simulink model "Closed_Loop_VC"  (R2016b)
settings: Solver=ode1  StartTime=0  StopTime=4  FixedStep=Time_Step  MaxStep=100e-6  RelTol=1e-3
undefined symbols (not defined in the file): Lg, Rg, Sn, Time_Step
libraries: powerlib x25, GFM_Lib x6, Source_Lib x2
settings Model: Creator=Frederic_Colas  LastModifiedBy=Frederic_Colas
settings OptimizationCC: LifeSpan=inf
settings DebuggingCC: UnconnectedInputMsg=none  UnconnectedOutputMsg=none  UnconnectedLineMsg=none  SFExecutionAtInitializationDiag=none
settings HardwareCC: ProdBitPerSizeT=32  ProdBitPerPtrDiffT=32  ProdWordSize=32  ProdHWDeviceType=Specified
settings SimscapeCC: SimscapeNormalizeSystem=off

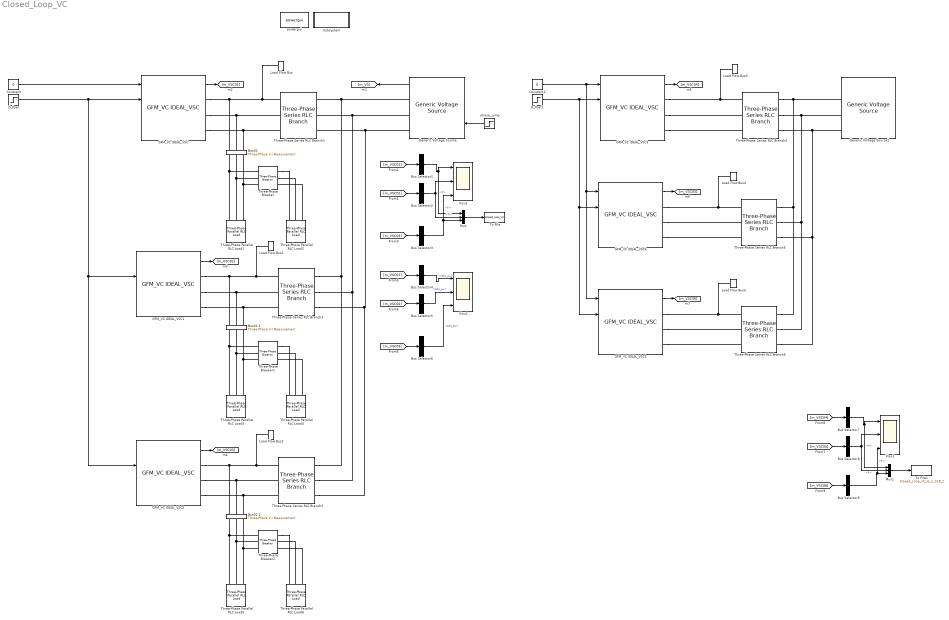
== system Closed_Loop_VC ==
  Bus Selector{1..3,7..9} (6 alike) : BusSelector  OutputSignals=P
  Bus Selector4 : BusSelector  OutputSignals=Ig.abc_pu
  Bus Selector5 : BusSelector  OutputSignals=Ig.abc_pu
  Bus Selector6 : BusSelector  OutputSignals=Ig.abc_pu
  "Bus02 " : powerlib/Measurements/Three-Phase V-I Measurement  VoltageMeasurement=no  SetLabelV=off  LabelV=Vabc  Vpu=off  VpuLL=off  CurrentMeasurement=no  SetLabelI=off  LabelI=Iabc  Ipu=off  Pbase=100e6  Vbase=500e3  OutputType=Complex  PhasorSimulation=off  PSBequivalent=0
  Bus02 1 : powerlib/Measurements/Three-Phase V-I Measurement  VoltageMeasurement=no  SetLabelV=off  LabelV=Vabc  Vpu=off  VpuLL=off  CurrentMeasurement=no  SetLabelI=off  LabelI=Iabc  Ipu=off  Pbase=100e6  Vbase=500e3  OutputType=Complex  PhasorSimulation=off  PSBequivalent=0
  Bus02 2 : powerlib/Measurements/Three-Phase V-I Measurement  VoltageMeasurement=no  SetLabelV=off  LabelV=Vabc  Vpu=off  VpuLL=off  CurrentMeasurement=no  SetLabelI=off  LabelI=Iabc  Ipu=off  Pbase=100e6  Vbase=500e3  OutputType=Complex  PhasorSimulation=off  PSBequivalent=0
  Constant : Constant  Value=0
  Constant1 : Constant  Value=0
  D_Pset : Step  Time=0.1  After=0.5  SampleTime=0
  D_Pset1 : Step  Time=0.1  After=0.5  SampleTime=0
  GFM_VC IDEAL_VSC : GFM_Lib/GFM_VC IDEAL_VSC  fn=fn  Sn=Sn  Pn=Sn  Udcn=640e3  Output_Delay=Time_Step  Un1=320e3  Un2=Un  Rt_pu=0.005  Lt_pu=0.15  Lm_pu=500  Rm_pu=500  DC_Link=Perfect DC Source  H_DC=inf  H_DC_sav=inf  wn_PLL=500  zeta_PLL=1  Val_Freq_Support=off  R_percent=4  dLc_pu=0  Rv=0.09  W_TVR=60  I_max_pu=1.2  wn_I_max=300  I_Max_TVI_pu=1.2  DX_DR=5  Advanced=off  gainpopup=Inertia Less  wn_Inertia_Less=10  Param_Inertia=PI  H_GFo=5  zeta_GFo=1  LFpopup=PQ  P0=0  Q0=0  V0=0.99839  Theta0=-0.85854
  GFM_VC IDEAL_VSC1 : GFM_Lib/GFM_VC IDEAL_VSC  fn=fn  Sn=Sn  Pn=Sn  Udcn=640e3  Output_Delay=Time_Step  Un1=320e3  Un2=Un  Rt_pu=0.005  Lt_pu=0.15  Lm_pu=500  Rm_pu=500  DC_Link=Perfect DC Source  H_DC=inf  H_DC_sav=inf  wn_PLL=50  zeta_PLL=1  Val_Freq_Support=off  R_percent=4  dLc_pu=0  Rv=0.09  W_TVR=60  I_max_pu=1.2  wn_I_max=300  I_Max_TVI_pu=1.2  DX_DR=5  Advanced=on  gainpopup=With Inertia  wn_Inertia_Less=10  Param_Inertia=VSM  H_GFo=5  zeta_GFo=1  LFpopup=PQ  P0=0  Q0=0  V0=0.99839  Theta0=-0.85854
  GFM_VC IDEAL_VSC2 : GFM_Lib/GFM_VC IDEAL_VSC  fn=fn  Sn=Sn  Pn=Sn  Udcn=640e3  Output_Delay=Time_Step  Un1=320e3  Un2=Un  Rt_pu=0.005  Lt_pu=0.15  Lm_pu=500  Rm_pu=500  DC_Link=Perfect DC Source  H_DC=inf  H_DC_sav=inf  wn_PLL=50  zeta_PLL=1  Val_Freq_Support=off  R_percent=4  dLc_pu=0  Rv=0.09  W_TVR=60  I_max_pu=1.2  wn_I_max=300  I_Max_TVI_pu=1.2  DX_DR=5  Advanced=on  gainpopup=With Inertia  wn_Inertia_Less=10  Param_Inertia=PI  H_GFo=5  zeta_GFo=1  LFpopup=PQ  P0=0  Q0=0  V0=0.99839  Theta0=-0.85854
  GFM_VC IDEAL_VSC3 : GFM_Lib/GFM_VC IDEAL_VSC  fn=fn  Sn=Sn  Pn=Sn  Udcn=640e3  Output_Delay=Time_Step  Un1=320e3  Un2=Un  Rt_pu=0.005  Lt_pu=0.15  Lm_pu=500  Rm_pu=500  DC_Link=Perfect DC Source  H_DC=inf  H_DC_sav=inf  wn_PLL=50  zeta_PLL=1  Val_Freq_Support=off  R_percent=4  dLc_pu=0  Rv=0.09  W_TVR=60  I_max_pu=1.2  wn_I_max=300  I_Max_TVI_pu=1.2  DX_DR=5  Advanced=on  gainpopup=With Inertia  wn_Inertia_Less=10  Param_Inertia=PI  H_GFo=5  zeta_GFo=1  LFpopup=PQ  P0=0  Q0=0  V0=1  Theta0=-3.2524e-13
  GFM_VC IDEAL_VSC4 : GFM_Lib/GFM_VC IDEAL_VSC  fn=fn  Sn=Sn  Pn=Sn  Udcn=640e3  Output_Delay=Time_Step  Un1=320e3  Un2=Un  Rt_pu=0.005  Lt_pu=0.15  Lm_pu=500  Rm_pu=500  DC_Link=Perfect DC Source  H_DC=inf  H_DC_sav=inf  wn_PLL=50  zeta_PLL=1  Val_Freq_Support=off  R_percent=4  dLc_pu=0  Rv=0.09  W_TVR=60  I_max_pu=1.2  wn_I_max=300  I_Max_TVI_pu=1.2  DX_DR=5  Advanced=on  gainpopup=With Inertia  wn_Inertia_Less=10  Param_Inertia=PI  H_GFo=1  zeta_GFo=1  LFpopup=PQ  P0=0  Q0=0  V0=1  Theta0=2.2332e-14
  GFM_VC IDEAL_VSC5 : GFM_Lib/GFM_VC IDEAL_VSC  fn=fn  Sn=Sn  Pn=Sn  Udcn=640e3  Output_Delay=Time_Step  Un1=320e3  Un2=Un  Rt_pu=0.005  Lt_pu=0.15  Lm_pu=500  Rm_pu=500  DC_Link=Perfect DC Source  H_DC=inf  H_DC_sav=inf  wn_PLL=50  zeta_PLL=1  Val_Freq_Support=off  R_percent=4  dLc_pu=0  Rv=0.09  W_TVR=60  I_max_pu=1.2  wn_I_max=300  I_Max_TVI_pu=1.2  DX_DR=5  Advanced=on  gainpopup=With Inertia  wn_Inertia_Less=10  Param_Inertia=PI  H_GFo=5  zeta_GFo=1  LFpopup=PQ  P0=0  Q0=0  V0=1  Theta0=2.2332e-14
  Generic Voltage Source : Source_Lib/Generic Voltage Source  SourceNature_str=INFINITE  fn=50  Sn=1e9  Un=400e3  H_s=5  DroopOnOff=on  R_percent=4  TN=1  TD=2  Time_Step=Time_Step  LFpopup=Swing  P0=898928563.4489  Q0=13470900.4169  V0=1  Theta0=0
  Generic Voltage Source1 : Source_Lib/Generic Voltage Source  SourceNature_str=INFINITE  fn=50  Sn=1e9  Un=400e3  H_s=5  DroopOnOff=on  R_percent=4  TN=1  TD=2  Time_Step=Time_Step  LFpopup=Swing  P0=3.3307e-06  Q0=7.1054e-06  V0=1  Theta0=0
  Load Flow Bus : powerlib/Measurements/Load Flow Bus  LConnTagsString=a  Phases=single  Connectors=on one side  ID=BUS_1  Vbase=400e3  Vref=1  Vangle=0  VLF=0.9984  VLFb=1  VLFc=1  angleLF=-0.8585  angleLFb=0  angleLFc=0
  Load Flow Bus1 : powerlib/Measurements/Load Flow Bus  LConnTagsString=a  Phases=single  Connectors=on one side  ID=BUS_2  Vbase=400e3  Vref=1  Vangle=0  VLF=0.9984  VLFb=1  VLFc=1  angleLF=-0.8585  angleLFb=0  angleLFc=0
  Load Flow Bus2 : powerlib/Measurements/Load Flow Bus  LConnTagsString=a  Phases=single  Connectors=on one side  ID=BUS_3  Vbase=400e3  Vref=1  Vangle=0  VLF=0.9984  VLFb=1  VLFc=1  angleLF=-0.8585  angleLFb=0  angleLFc=0
  Load Flow Bus3 : powerlib/Measurements/Load Flow Bus  LConnTagsString=a  Phases=single  Connectors=on one side  ID=BUS_4  Vbase=400e3  Vref=1  Vangle=0  VLF=1  VLFb=1  VLFc=1  angleLF=-3.252e-13  angleLFb=0  angleLFc=0
  Load Flow Bus4 : powerlib/Measurements/Load Flow Bus  LConnTagsString=a  Phases=single  Connectors=on one side  ID=BUS_5  Vbase=400e3  Vref=1  Vangle=0  VLF=1  VLFb=1  VLFc=1  angleLF=2.233e-14  angleLFb=0  angleLFc=0
  Load Flow Bus5 : powerlib/Measurements/Load Flow Bus  LConnTagsString=a  Phases=single  Connectors=on one side  ID=BUS_6  Vbase=400e3  Vref=1  Vangle=0  VLF=1  VLFb=1  VLFc=1  angleLF=2.233e-14  angleLFb=0  angleLFc=0
  Mux : Mux  Inputs=3
  Mux1 : Mux  Inputs=3
  Subsystem : Subsystem
      settings: OpenFcn=LoadFlow_VSC
      mask Display: color('blue'),disp('Update Loadflow')
  Three-Phase Parallel RLC Load1 : powerlib/Elements/Three-Phase Parallel RLC Load  LConnTagsString=A|B|C  Configuration=Y (grounded)  NominalVoltage=Un  Vabc=[1e3 1e3 1e3]  Vabcp=[1e3 1e3 1e3]  NominalFrequency=fn  UnbalancedPower=off  ActivePower=0.3*Sn  InductivePower=0  CapacitivePower=0  Pabc=[10e3 9e3 11e3]  QLabc=[100 90 110]  QCabc=[100 90 110]  Pabcp=[10e3 9e3 11e3]  QLabcp=[100 90 110]  QCabcp=[100 90 110]  Measurements=None  LoadType=constant Z
  Three-Phase Parallel RLC Load2 : powerlib/Elements/Three-Phase Parallel RLC Load  LConnTagsString=A|B|C  Configuration=Y (grounded)  NominalVoltage=Un  Vabc=[1e3 1e3 1e3]  Vabcp=[1e3 1e3 1e3]  NominalFrequency=fn  UnbalancedPower=off  ActivePower=0.5*Sn  InductivePower=0  CapacitivePower=0  Pabc=[10e3 9e3 11e3]  QLabc=[100 90 110]  QCabc=[100 90 110]  Pabcp=[10e3 9e3 11e3]  QLabcp=[100 90 110]  QCabcp=[100 90 110]  Measurements=None  LoadType=constant Z
  Three-Phase Parallel RLC Load3 : powerlib/Elements/Three-Phase Parallel RLC Load  LConnTagsString=A|B|C  Configuration=Y (grounded)  NominalVoltage=Un  Vabc=[1e3 1e3 1e3]  Vabcp=[1e3 1e3 1e3]  NominalFrequency=fn  UnbalancedPower=off  ActivePower=0.3*Sn  InductivePower=0  CapacitivePower=0  Pabc=[10e3 9e3 11e3]  QLabc=[100 90 110]  QCabc=[100 90 110]  Pabcp=[10e3 9e3 11e3]  QLabcp=[100 90 110]  QCabcp=[100 90 110]  Measurements=None  LoadType=constant Z
  Three-Phase Parallel RLC Load4 : powerlib/Elements/Three-Phase Parallel RLC Load  LConnTagsString=A|B|C  Configuration=Y (grounded)  NominalVoltage=Un  Vabc=[1e3 1e3 1e3]  Vabcp=[1e3 1e3 1e3]  NominalFrequency=fn  UnbalancedPower=off  ActivePower=0.5*Sn  InductivePower=0  CapacitivePower=0  Pabc=[10e3 9e3 11e3]  QLabc=[100 90 110]  QCabc=[100 90 110]  Pabcp=[10e3 9e3 11e3]  QLabcp=[100 90 110]  QCabcp=[100 90 110]  Measurements=None  LoadType=constant Z
  Three-Phase Parallel RLC Load5 : powerlib/Elements/Three-Phase Parallel RLC Load  LConnTagsString=A|B|C  Configuration=Y (grounded)  NominalVoltage=Un  Vabc=[1e3 1e3 1e3]  Vabcp=[1e3 1e3 1e3]  NominalFrequency=fn  UnbalancedPower=off  ActivePower=0.3*Sn  InductivePower=0  CapacitivePower=0  Pabc=[10e3 9e3 11e3]  QLabc=[100 90 110]  QCabc=[100 90 110]  Pabcp=[10e3 9e3 11e3]  QLabcp=[100 90 110]  QCabcp=[100 90 110]  Measurements=None  LoadType=constant Z
  Three-Phase Parallel RLC Load6 : powerlib/Elements/Three-Phase Parallel RLC Load  LConnTagsString=A|B|C  Configuration=Y (grounded)  NominalVoltage=Un  Vabc=[1e3 1e3 1e3]  Vabcp=[1e3 1e3 1e3]  NominalFrequency=fn  UnbalancedPower=off  ActivePower=0.5*Sn  InductivePower=0  CapacitivePower=0  Pabc=[10e3 9e3 11e3]  QLabc=[100 90 110]  QCabc=[100 90 110]  Pabcp=[10e3 9e3 11e3]  QLabcp=[100 90 110]  QCabcp=[100 90 110]  Measurements=None  LoadType=constant Z
  Three-Phase Series RLC Branch{1..3,5..6} (5 alike) : powerlib/Elements/Three-Phase Series RLC Branch  LConnTagsString=A|B|C  RConnTagsString=A|B|C  BranchType=RL  Resistance=Rg  Inductance=Lg  Capacitance=1e-6  Measurements=None
  Three-Phase Series RLC Branch4 : powerlib/Elements/Three-Phase Series RLC Branch  LConnTagsString=A|B|C  RConnTagsString=A|B|C  BranchType=RL  Resistance=Rg*10  Inductance=Lg*10  Capacitance=1e-6  Measurements=None
  Three-Phase Breaker : powerlib/Elements/Three-Phase Breaker  InitialState=open  SwitchA=on  SwitchB=on  SwitchC=on  SwitchTimes=10  External=off  BreakerResistance=0.01  SnubberResistance=1e6  SnubberCapacitance=inf  Measurements=None
  Three-Phase Breaker1 : powerlib/Elements/Three-Phase Breaker  InitialState=open  SwitchA=on  SwitchB=on  SwitchC=on  SwitchTimes=10  External=off  BreakerResistance=0.01  SnubberResistance=1e6  SnubberCapacitance=inf  Measurements=None
  Three-Phase Breaker2 : powerlib/Elements/Three-Phase Breaker  InitialState=open  SwitchA=on  SwitchB=on  SwitchC=on  SwitchTimes=10  External=off  BreakerResistance=0.01  SnubberResistance=1e6  SnubberCapacitance=inf  Measurements=None
  To File : ToFile  Filename=Closed_Loop_VC  MatrixName=power  SaveFormat=Timeseries
  To File1 : ToFile  Filename=Closed_Loop_VC_H_1_SCR_2  MatrixName=power  SaveFormat=Timeseries
  Visu1 : Scope  NumInputPorts=3
  Visu2 : Scope  NumInputPorts=3
  Visu3 : Scope  NumInputPorts=3
  phase_jump : Step  After=pi/40  SampleTime=0
  powergui : powerlib/powergui  Priority=1  SimulationMode=Discrete  SampleTime=Time_Step  frequency=60  Iterations=50  frequencyindice=50  Pbase=1000000000  ErrMax=1e-6  UnitsV=kV  UnitsW=MW  buscounter=0  FunctionMessages=off  echomessages=off  EnableUseOfTLC=off  CurrentSourceSwitches=off  DisableSnubberDevices=off  DisableRonSwitches=off  DisableVfSwitches=off  DisplayEquations=off  AutomaticDiscreteSolvers=off  SolverType=Tustin/Backward Euler (TBE)  Interpol=off  ExternalGateDelay=off  methode=off  Ts=100  x0status=blocks  SPID=on  SwTol=0  HookPort=off  NonlinearTolerance=1e-4  nMaxIteration=100  ContinueOnMaxIteration=off  RestoreLinks=warning  ResistiveCurrentMeasurement=off  Frange=[0:2:500]  Ylog=off  Xlog=on  ShowGrid=off  save=off  variable=ZData  structure=0  ZoomFFT=off  StartTime=0.0  cycles=1  DisplayStyle=1  fundamental=60  FreqAxis=off  MaxFrequency=1000  frequencyindicesteady=1  RmsSteady=1  display=off
  wires:
  Constant/1 -> GFM_VC IDEAL_VSC/1
  Generic Voltage Source/1 -> [m_VS]
  D_Pset/1 -> GFM_VC IDEAL_VSC2/2, GFM_VC IDEAL_VSC1/2, GFM_VC IDEAL_VSC/2
  phase_jump/1 -> Generic Voltage Source/2
  [m_VSC01] -> Bus Selector1/1
  GFM_VC IDEAL_VSC/1 -> [m_VSC01]
  Bus Selector1/1 -> Mux/1, Visu1/1  "<P>"
  GFM_VC IDEAL_VSC1/1 -> [m_VSC02]
  [m_VSC02] -> Bus Selector2/1
  Bus Selector2/1 -> Mux/2, Visu1/2  "<P>"
  Mux/1 -> To File/1
  GFM_VC IDEAL_VSC2/1 -> [m_VSC03]
  [m_VSC03] -> Bus Selector3/1
  Bus Selector3/1 -> Mux/3, Visu1/3  "<P>"
  Bus Selector6/1 -> Visu2/3  "<abc_pu>"
  [m_VSC03] -> Bus Selector6/1
  Bus Selector5/1 -> Visu2/2  "<abc_pu>"
  [m_VSC02] -> Bus Selector5/1
  Bus Selector4/1 -> Visu2/1  "<abc_pu>"
  [m_VSC01] -> Bus Selector4/1
  GFM_VC IDEAL_VSC3/1 -> [m_VSC04]
  GFM_VC IDEAL_VSC4/1 -> [m_VSC05]
  Constant1/1 -> GFM_VC IDEAL_VSC5/1, GFM_VC IDEAL_VSC4/1, GFM_VC IDEAL_VSC3/1
  D_Pset1/1 -> GFM_VC IDEAL_VSC5/2, GFM_VC IDEAL_VSC4/2, GFM_VC IDEAL_VSC3/2
  Mux1/1 -> To File1/1
  Bus Selector8/1 -> Visu3/2, Mux1/2  "<P>"
  [m_VSC05] -> Bus Selector8/1
  Bus Selector7/1 -> Visu3/1, Mux1/1  "<P>"
  [m_VSC04] -> Bus Selector7/1
  GFM_VC IDEAL_VSC5/1 -> [m_VSC06]
  [m_VSC06] -> Bus Selector9/1
  Bus Selector9/1 -> Visu3/3, Mux1/3  "<P>"
  connections:
  "Bus02 "/LConn3 -- GFM_VC IDEAL_VSC/RConn1 -- Load Flow Bus/LConn1 -- Three-Phase Series RLC Branch1/LConn1
  "Bus02 "/LConn1 -- GFM_VC IDEAL_VSC/RConn3 -- Three-Phase Series RLC Branch1/LConn3
  "Bus02 "/LConn2 -- GFM_VC IDEAL_VSC/RConn2 -- Three-Phase Series RLC Branch1/LConn2
  Generic Voltage Source/RConn1 -- Three-Phase Series RLC Branch3/RConn1 -- Three-Phase Series RLC Branch2/RConn1 -- Three-Phase Series RLC Branch1/RConn1
  Generic Voltage Source/RConn2 -- Three-Phase Series RLC Branch3/RConn2 -- Three-Phase Series RLC Branch2/RConn2 -- Three-Phase Series RLC Branch1/RConn2
  Generic Voltage Source/RConn3 -- Three-Phase Series RLC Branch3/RConn3 -- Three-Phase Series RLC Branch2/RConn3 -- Three-Phase Series RLC Branch1/RConn3
  "Bus02 "/RConn1 -- Three-Phase Breaker/LConn3 -- Three-Phase Parallel RLC Load1/LConn3
  "Bus02 "/RConn2 -- Three-Phase Breaker/LConn2 -- Three-Phase Parallel RLC Load1/LConn2
  "Bus02 "/RConn3 -- Three-Phase Breaker/LConn1 -- Three-Phase Parallel RLC Load1/LConn1
  Three-Phase Parallel RLC Load2/LConn2 -- Three-Phase Breaker/RConn2
  Three-Phase Breaker/RConn1 -- Three-Phase Parallel RLC Load2/LConn1
  Three-Phase Parallel RLC Load2/LConn3 -- Three-Phase Breaker/RConn3
  Three-Phase Series RLC Branch2/LConn1 -- Bus02 1/LConn3 -- GFM_VC IDEAL_VSC1/RConn1 -- Load Flow Bus1/LConn1
  GFM_VC IDEAL_VSC1/RConn2 -- Three-Phase Series RLC Branch2/LConn2 -- Bus02 1/LConn2
  GFM_VC IDEAL_VSC1/RConn3 -- Three-Phase Series RLC Branch2/LConn3 -- Bus02 1/LConn1
  Three-Phase Parallel RLC Load3/LConn1 -- Bus02 1/RConn3 -- Three-Phase Breaker1/LConn1
  Three-Phase Parallel RLC Load3/LConn2 -- Bus02 1/RConn2 -- Three-Phase Breaker1/LConn2
  Three-Phase Parallel RLC Load3/LConn3 -- Bus02 1/RConn1 -- Three-Phase Breaker1/LConn3
  Three-Phase Parallel RLC Load4/LConn2 -- Three-Phase Breaker1/RConn2
  Three-Phase Parallel RLC Load4/LConn3 -- Three-Phase Breaker1/RConn3
  Three-Phase Breaker1/RConn1 -- Three-Phase Parallel RLC Load4/LConn1
  Three-Phase Parallel RLC Load5/LConn1 -- Bus02 2/RConn3 -- Three-Phase Breaker2/LConn1
  Three-Phase Parallel RLC Load5/LConn2 -- Bus02 2/RConn2 -- Three-Phase Breaker2/LConn2
  GFM_VC IDEAL_VSC2/RConn2 -- Three-Phase Series RLC Branch3/LConn2 -- Bus02 2/LConn2
  GFM_VC IDEAL_VSC2/RConn3 -- Three-Phase Series RLC Branch3/LConn3 -- Bus02 2/LConn1
  Load Flow Bus2/LConn1 -- Bus02 2/LConn3 -- GFM_VC IDEAL_VSC2/RConn1 -- Three-Phase Series RLC Branch3/LConn1
  Three-Phase Parallel RLC Load5/LConn3 -- Bus02 2/RConn1 -- Three-Phase Breaker2/LConn3
  Three-Phase Parallel RLC Load6/LConn3 -- Three-Phase Breaker2/RConn3
  Three-Phase Parallel RLC Load6/LConn2 -- Three-Phase Breaker2/RConn2
  Three-Phase Breaker2/RConn1 -- Three-Phase Parallel RLC Load6/LConn1
  Three-Phase Series RLC Branch4/LConn1 -- GFM_VC IDEAL_VSC3/RConn1 -- Load Flow Bus3/LConn1
  GFM_VC IDEAL_VSC3/RConn2 -- Three-Phase Series RLC Branch4/LConn2
  GFM_VC IDEAL_VSC3/RConn3 -- Three-Phase Series RLC Branch4/LConn3
  Three-Phase Series RLC Branch4/RConn1 -- Three-Phase Series RLC Branch6/RConn1 -- Three-Phase Series RLC Branch5/RConn1 -- Generic Voltage Source1/RConn1
  Three-Phase Series RLC Branch4/RConn2 -- Three-Phase Series RLC Branch6/RConn2 -- Three-Phase Series RLC Branch5/RConn2 -- Generic Voltage Source1/RConn2
  Three-Phase Series RLC Branch4/RConn3 -- Three-Phase Series RLC Branch6/RConn3 -- Three-Phase Series RLC Branch5/RConn3 -- Generic Voltage Source1/RConn3
  GFM_VC IDEAL_VSC4/RConn1 -- Three-Phase Series RLC Branch5/LConn1 -- Load Flow Bus4/LConn1
  GFM_VC IDEAL_VSC4/RConn2 -- Three-Phase Series RLC Branch5/LConn2
  GFM_VC IDEAL_VSC4/RConn3 -- Three-Phase Series RLC Branch5/LConn3
  Three-Phase Series RLC Branch6/LConn1 -- GFM_VC IDEAL_VSC5/RConn1 -- Load Flow Bus5/LConn1
  GFM_VC IDEAL_VSC5/RConn2 -- Three-Phase Series RLC Branch6/LConn2
  GFM_VC IDEAL_VSC5/RConn3 -- Three-Phase Series RLC Branch6/LConn3

== system Closed_Loop_VC/Subsystem ==
